simulink library "InfrastructureVariants_CL"  (R2020a)
settings: Solver=VariableStepAuto  StartTime=0.0  StopTime=10.0  RelTol=1e-3
undefined symbols (not defined in the file): Buffer, ENV, Int, Int_ran, route, TRAN, VEH
(part 2 of 2)

== matlab function InfrastructureVariants_CL/Infrastructure v0/Signal Info v5/Cycle v5 ==
  data: Sig_out output; Int_out output; t_0 input; Sig_in input; Int_in input; hyp_out output; hyp input; Buffer input
function [Sig_out,Int_out,hyp_out] = fcn(t_0,Sig_in,Int_in,hyp,Buffer)

Int_cur = Int_in(~isnan(Int_in(:,1)),1);        %   Current intersections within communication range
Cs = Sig_in(:,:,1);                             %   s - Signal cycle start times
G = Sig_in(:,:,3);                              %   s - Signal green phase length 
R = Sig_in(:,:,4);                              %   s - Signal red phase length 
Y = Buffer(:,1);                                %   s - Signal yellow length
Rc = Buffer(:,2);                               %   s - Signal red clearance length 
N = 10;                                         %   # of upcoming intersections 
M = 20;                                         %   Size of intersection data queue
idx = zeros(N,1);                               %   Initialize current cycle index vector
Sig_out = NaN*ones(N,M,4);                      %   Initialize cycle length output 
hyp_out = NaN*ones(N,3,2);                      %   Initialize hyperparameter output 
T_0 = NaN*ones(N,1);                            %   Initialize current cycle start time output
L_0 = NaN*ones(N,1);                            %   Initialize light status flag
B_0 = NaN*ones(N,1);                            %   Initialize yellow light length 
for i = 1:length(Int_cur)
    idx(i) = find(Cs(Int_cur(i),:) <= t_0,1,'last');        %   Find current cycle for upcoming intersections 
    tR = Cs(Int_cur(i),idx(i))+G(Int_cur(i),idx(i));        %   s - Time at which light turns red
    tL1 = tR-t_0;                                           %   s - Time left until red
    tL2 = Cs(Int_cur(i),idx(i)+1)-t_0;                      %   s - Time left until green
    if tL1 > Y(Int_cur(i))*2 
        L_0(i) = 0;                                         %   Light is green and time left is unknown 
        Sig_out(i,:,3) = idx(i)-M:idx(i)-1;                 %   Available green phase lengths
        Sig_out(i,:,4) = idx(i)-M:idx(i)-1;                 %   Available red phase lengths
    elseif tL1 <= Y(Int_cur(i))*2 && tL1 > 0
        L_0(i) = 1;                                         %   Light is green and time left is known 
        Sig_out(i,:,3) = idx(i)-M+1:idx(i);                 %   Available green phase lengths
        Sig_out(i,:,4) = idx(i)-M:idx(i)-1;                 %   Available red phase lengths
    elseif tL2 > (Y(Int_cur(i))+Rc(Int_cur(i)))*2 
        L_0(i) = 2;                                         %   Light is red and time left is unknown 
        Sig_out(i,:,3) = idx(i)-M+1:idx(i);                 %   Available green phase lengths
        Sig_out(i,:,4) = idx(i)-M:idx(i)-1;                 %   Available red phase lengths
    else           
        L_0(i) = 3;                                         %   Light is red and time left is known 
        Sig_out(i,:,3) = idx(i)-M+1:idx(i);                 %   Available green phase lengths
        Sig_out(i,:,4) = idx(i)-M+1:idx(i);                 %   Available red phase lengths
    end
    B_0(i) = 2*Y(Int_cur(i));                               %   Yellow light length for upcoming intersections 
    Sig_out(i,:,1) = G(Int_cur(i),Sig_out(i,:,3));          %   Create a vector with the past green phase lengths
    Sig_out(i,:,2) = R(Int_cur(i),Sig_out(i,:,4));          %   Create a vector with the past red phase lengths
    T_0(i) = Cs(Int_cur(i),idx(i));                         %   Current cycle start time
    hypG1 = var(Sig_out(i,:,1));
    hypR1 = var(Sig_out(i,:,2));
    hyp_out(i,:,1) = [hypG1 1 .0625];                       %   Get relevant hyperparameters 
    hyp_out(i,:,2) = [hypR1 1 .0625];                       %   Get relevant hyperparameters 
end
Int_out = [Int_in, T_0, L_0, B_0];                          %   Update intersection variables

== matlab function InfrastructureVariants_CL/Infrastructure v0/Signal Info v5/IntFcn ==
  data: x_0 input; I_mode output; Int_ran input; Int_pos input; Int_out output
function [I_mode,Int_out]  = fcn(x_0,Int_ran,Int_pos)

Int_pos = Int_pos(:,1);                         %   Intersection Positions
[Int_0,~] = find(x_0-Int_pos < 0,1,'first');    %   First intersection within range
[Int_f,~] = find(x_0+Int_ran-Int_pos...         %   Last intersection within range
    > 0,1,'last');
Int_cur = NaN*ones(10,1);                       %   Initialize upcoming intersection vector 
Int_dx = NaN*ones(10,1);                        %   m - Initialize distance to upcoming intersections vector 
Int_gap = NaN*ones(10,1);                       %   m - Initialize distance between intersections vector 
if isempty(Int_0)
    I_mode = 0;                                 %   No upcoming intersection
elseif Int_pos(Int_0(1))-x_0 > Int_ran
    I_mode = 0;                                 %   No upcoming intersection
else
    I_0 = Int_0(1);     I_f = Int_f(1);
    Int_cur(1:I_f-I_0+1,1) = (I_0:I_f)';            %   Upcoming intersections
    I_mode = 1;                                 %   Approaching intersection
    Int_dx(1:I_f-I_0+1,1) = ...                 %   m - Distance to upcoming intersection 
        Int_pos(Int_cur(1:I_f-I_0+1,1))-x_0;
end
Int_gap(1) = Int_dx(1);                         %   m - Distance to first upcoming intersection 
for i = 2:length(Int_gap)
    Int_gap(i) = Int_dx(i)-Int_dx(i-1);         %   m - Distance between further intersections 
end
Int_out = [Int_cur,Int_dx,Int_gap];
